simulink model "part1"  (R2018a)
settings: Solver=VariableStepAuto  StartTime=0.0  StopTime=10.0  RelTol=1e-3
libraries: truetime x1
settings Model: Creator=Ismael  LastModifiedBy=Ismael

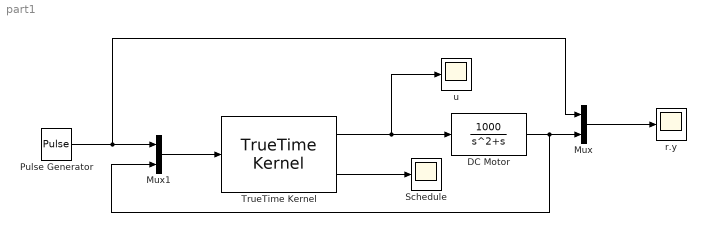
== system part1 ==
  DC Motor : TransferFcn  Numerator=[1000]  Denominator=[1 1 0]
  Mux : Mux  Inputs=2
  Mux1 : Mux  Inputs=2
  "Pulse Generator " : DiscretePulseGenerator  PulseType=Time based  Amplitude=2  Period=1  PulseWidth=50  PhaseDelay=0.1
  Schedule : Scope
  "TrueTime Kernel " : truetime/TrueTime Kernel  sfun=part1_init  args=0.005  ninputsoutputs=[2 1]  ntriggers=0  trigtype=falling  nwnodenbr=[]  clockoffsetdrift=[0 0]  schedoutput=on  battery=off  poweroutput=off
  r.y : Scope
  u : Scope
  wires:
  "TrueTime Kernel "/1 -> DC Motor/1, u/1
  "TrueTime Kernel "/2 -> Schedule/1
  DC Motor/1 -> Mux1/2, Mux/2
  Mux/1 -> r.y/1
  Mux1/1 -> "TrueTime Kernel "/1
  "Pulse Generator "/1 -> Mux/1, Mux1/1
